simulink model "DLHnguoc3DOF"  (R2020b)
settings: Solver=VariableStepAuto  StartTime=0.0  StopTime=10.0  RelTol=1e-3
settings Model: Creator=Dell  LastModifiedBy=Nothing
settings DataIOCC: ReturnWorkspaceOutputs=off
settings DebuggingCC: ArithmeticOperatorsInVariantConditions=warning
settings SFSimCC: SimUseLocalCustomCode=off  CustomCodeUndefinedFunction=UseInterfaceOnly
settings RTWCC: RTWUseLocalCustomCode=off
settings CodeAppCC: StateflowObjectComments=on

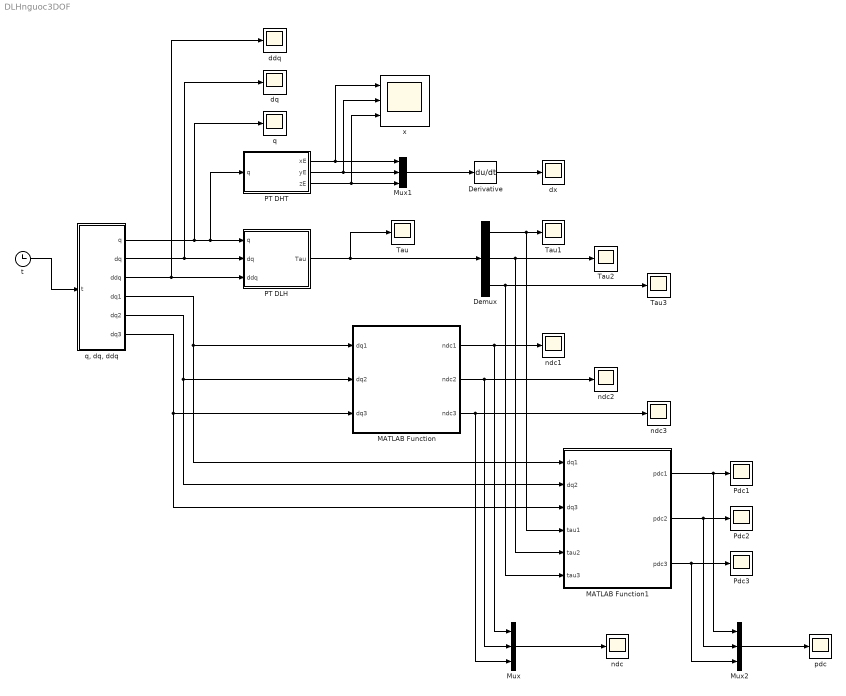
== system DLHnguoc3DOF ==
  Demux : Demux  Outputs=3
  Derivative : Derivative
  MATLAB Function : MATLAB Function  TreatAsAtomicUnit=on
  MATLAB Function1 : MATLAB Function  TreatAsAtomicUnit=on
  Mux : Mux  Inputs=3
  Mux1 : Mux  Inputs=3
  Mux2 : Mux  Inputs=3
  PT DHT : MATLAB Function  TreatAsAtomicUnit=on
  PT DLH : MATLAB Function  TreatAsAtomicUnit=on
  Pdc1 : Scope
  Pdc2 : Scope
  Pdc3 : Scope
  Tau{,1..3} (4 alike) : Scope
  ddq : Scope
  dq : Scope
  dx : Scope
  ndc{,1..3} (4 alike) : Scope
  pdc : Scope
  q : Scope
  "q, dq, ddq" : MATLAB Function  TreatAsAtomicUnit=on
  t : Clock
  x : Scope  NumInputPorts=3
  wires:
  "q, dq, ddq"/1(q) -> PT DHT/1(q), PT DLH/1(q), q/1
  t/1 -> "q, dq, ddq"/1(t)
  "q, dq, ddq"/2(dq) -> dq/1, PT DLH/2(dq)
  "q, dq, ddq"/3(ddq) -> ddq/1, PT DLH/3(ddq)
  PT DLH/1(Tau) -> Demux/1, Tau/1
  PT DHT/2(yE) -> x/2, Mux1/2
  PT DHT/3(zE) -> x/3, Mux1/3
  PT DHT/1(xE) -> x/1, Mux1/1
  Mux1/1 -> Derivative/1
  Derivative/1 -> dx/1
  Demux/1 -> MATLAB Function1/4(tau1), Tau1/1
  Demux/2 -> MATLAB Function1/5(tau2), Tau2/1
  Demux/3 -> MATLAB Function1/6(tau3), Tau3/1
  "q, dq, ddq"/4(dq1) -> MATLAB Function/1(dq1), MATLAB Function1/1(dq1)
  "q, dq, ddq"/5(dq2) -> MATLAB Function1/2(dq2), MATLAB Function/2(dq2)
  "q, dq, ddq"/6(dq3) -> MATLAB Function/3(dq3), MATLAB Function1/3(dq3)
  MATLAB Function1/1(pdc1) -> Mux2/1, Pdc1/1
  MATLAB Function1/2(pdc2) -> Mux2/2, Pdc2/1
  MATLAB Function1/3(pdc3) -> Mux2/3, Pdc3/1
  MATLAB Function/1(ndc1) -> Mux/1, ndc1/1
  MATLAB Function/2(ndc2) -> Mux/2, ndc2/1
  MATLAB Function/3(ndc3) -> Mux/3, ndc3/1
  Mux/1 -> ndc/1
  Mux2/1 -> pdc/1

== matlab function DLHnguoc3DOF/PT DLH ==
  data: q input; Tau output; dq input; ddq input
function Tau  =DLHN(q,dq,ddq)
[m1,m2,m3,L1,L2,L3,I1x,I1y,I1z,I2x,I2y,I2z,I3x,I3y,I3z]=parameter ();

% Khai bao ma tran khoi luong M
M=zeros(3,3);
M(1,1)= (9/4)*m1*L1^2+I1z+3*m2*L2*L1*cos(q(2))+L1^2*m2+(9/4)*m2*L2^2+I2y+2*m3*L2*L1*cos(q(2))+3*m3*L1*q(3)*sin(q(2))+L1^2*m3+L2^2*m3+(9/4)*m3*q(3)^2+I3y;
M(1,2)= (3/2)*m2*L2*L1*cos(q(2))+(9/4)*m2*L2^2+I2y+m3*L2*L1*cos(q(2))+(3/2)*m3*L1*q(3)*sin(q(2))+L2^2*m3+(9/4)*m3*q(3)^2+I3y;
M(1,3)= -(3/2)*L1*m3*cos(q(2))-(3/2)*L2*m3;


M(2,1)=(3/2)*m2*L2*L1*cos(q(2))+(9/4)*m2*L2^2+I2y+m3*L2*L1*cos(q(2))+(3/2)*m3*L1*q(3)*sin(q(2))+L2^2*m3+(9/4)*m3*q(3)^2+I3y;
M(2,2)=(9/4)*m2*L2^2+I2y+L2^2*m3+(9/4)*m3*q(3)^2+I3y;
M(2,3)=-(3/2)*L2*m3;

M(3,1)=-(3/2)*L1*m3*cos(q(2))-(3/2)*L2*m3;
M(3,2)=-(3/2)*L2*m3;
M(3,3)=(9/4)*m3;

% Khai bao ma tran Coriolis C
%h=-m2*L1*Lc2*sin(q(2));
Co=zeros(3,3);
Co(1,1)=-3*L1*L2*sin(q(2))*dq(2)*m2-2*L1*L2*sin(q(2))*dq(2)*m3+3*L1*cos(q(2))*dq(2)*m3*q(3)+3*L1*m3*sin(q(2))*dq(3)+(9/2)*m3*q(3)*dq(3);
Co(1,2)=-(3/2)*L1*L2*sin(q(2))*dq(2)*m2-L1*L2*sin(q(2))*dq(2)*m3+(3/2)*L1*cos(q(2))*dq(2)*m3*q(3)+(3/2)*L1*m3*sin(q(2))*dq(3)+(9/2)*m3*q(3)*dq(3);
Co(1,3)=(3/2)*L1*m3*sin(q(2))*dq(2);


Co(2,1)=(3/2)*L1*L2*sin(q(2))*dq(1)*m2+L1*L2*sin(q(2))*dq(1)*m3-(3/4)*L1*L2*sin(q(2))*dq(2)*m2-(1/2)*L1*L2*sin(q(2))*dq(2)*m3-(3/2)*L1*cos(q(2))*dq(1)*m3*q(3)+(3/4)*L1*cos(q(2))*dq(2)*m3*q(3)+(3/4)*L1*m3*sin(q(2))*dq(3)+(9/2)*m3*q(3)*dq(3);
Co(2,2)=(3/4)*L1*L2*sin(q(2))*dq(1)*m2+(1/2)*L1*L2*sin(q(2))*dq(1)*m3-(3/4)*L1*cos(q(2))*dq(1)*m3*q(3)+(9/2)*m3*q(3)*dq(3);
Co(2,3)=-(3/4)*L1*m3*sin(q(2))*dq(1);


Co(3,1)=-(3/2)*L1*m3*sin(q(2))*dq(1)+(3/4)*L1*m3*sin(q(2))*dq(2)-(9/4)*dq(1)*m3*q(3)-(9/4)*m3*q(3)*dq(2);
Co(3,2)=-(3/4)*L1*m3*sin(q(2))*dq(1)-(9/4)*dq(1)*m3*q(3)-(9/4)*m3*q(3)*dq(2);
Co(3,3)=0;

% Ma tran the nang hap dan
G=zeros(3,1);
G(1,1)=15*m1*L1*cos(q(1))+10*m2*L1*cos(q(1))+10*m3*L1*cos(q(1))+15*m2*L2*cos(q(1)+q(2))+10*m3*L2*cos(q(1)+q(2))+15*m3*sin(q(1)+q(2))*q(3);
G(2,1)=15*m2*L2*cos(q(1)+q(2))+10*m3*L2*cos(q(1)+q(2))+15*m3*sin(q(1)+q(2))*q(3);
G(3,1)=-15*m3*cos(q(1)+q(2));


% Pt DLH
Tau=M*ddq + Co*dq + G;

== matlab function DLHnguoc3DOF/q, dq, ddq ==
  data: q output; t input; dq output; ddq output; dq1 output; dq2 output; dq3 output
function [q,dq,ddq,dq1,dq2,dq3] = fcn(t)
Pi=3.14;
q1 = (1/3)*Pi-(1/400)*t^2*Pi+(1/6000)*t^3*Pi;
q2 = (1/6)*Pi-(1/500)*t^2*Pi+(1/7500)*t^3*Pi;
q3 = 0.2-0.003*t^2+0.0002*t^3;

q=zeros(3,1);
q(1,1)=q1;
q(2,1)=q2;
q(3,1)=q3;

dq1=-(1/200)*t*Pi+(1/2000)*t^2*Pi;
dq2=-(1/250)*t*Pi+(1/2500)*t^2*Pi;
dq3=-0.006*t+0.0006*t^2;

dq=zeros(3,1);
dq(1,1)=dq1;
dq(2,1)=dq2;
dq(3,1)=dq3;

ddq1=-(1/200)*Pi+(1/1000)*t*Pi;
ddq2=-(1/250)*Pi+(1/1250)*t*Pi;
ddq3=-0.006+0.0012*t;

ddq=zeros(3,1);
ddq(1,1)=ddq1;
ddq(2,1)=ddq2;
ddq(3,1)=ddq3;

== matlab function DLHnguoc3DOF/PT DHT ==
  data: xE output; q input; yE output; zE output
function [xE,yE,zE] = fcn(q)
[m1,m2,m3,L1,L2,L3,I1x,I1y,I1z,I2x,I2y,I2z,I3x,I3y,I3z]=parameter ();
q1=q(1,1);
q2=q(2,1);
q3=q(3,1);
xE = sin(q1+q2)*q3+L2*cos(q1+q2)+L1*cos(q1);
yE = -cos(q1+q2)*q3+L2*sin(q1+q2)+L1*sin(q1);
zE = 0;

== matlab function DLHnguoc3DOF/MATLAB Function ==
  data: dq1 input; ndc1 output; dq2 input; dq3 input; ndc2 output; ndc3 output
function [ndc1,ndc2,ndc3] = Tinhvongquaydongco(dq1,dq2,dq3)

ndc1=(dq1*60)/(2*pi);
ndc2=(dq2*60)/(2*pi);
ndc3=(dq3*60)/(2*pi);

== matlab function DLHnguoc3DOF/MATLAB Function1 ==
  data: dq1 input; pdc1 output; dq2 input; dq3 input; pdc2 output; pdc3 output; tau1 input; tau2 input; tau3 input
function [pdc1,pdc2,pdc3] = Tinhcongsuatdongco(dq1,dq2,dq3,tau1,tau2,tau3)
nuy=0.95; % Hieu suat lam viec
plv1=tau1*dq1/1000;
plv2=tau2*dq2/1000;
plv3=tau3*dq3/1000;

pdc1=plv1/nuy;
pdc2=plv2/nuy;
pdc3=plv3/nuy;
